simulink model "Simulink_Arduino_PIL_v05"  (R2020a)
settings: Solver=VariableStepAuto  StartTime=0.0  StopTime=Tsim  RelTol=1e-3
values from neighbouring files (symbols this model uses):
  A = [0.637125393971 0.00050275765043 2.56129190029e-05 0.00322036092898 7.22167712685e-07 3.54290406932e-08 0.00050275765043 0.637125393971 -2.56129190029e-05 7.22167712685e-07 0.00322036092898 -3.54290406932e-08 ... (36 elements, 6x6)]    [exitationData.mat]    (also in main_Simulink_Arduino_PIL_v05.m = sys_dt.A; main_Simulink_Arduino_PIL_v05_v2.m = SSDClip.A; result_data.mat = [0.828490331528 0.231089081296 -0.073917292718 -0.1174239001)
  Ac = [-112.5 0 0 1 0 0 0 -112.5 0 0 1 0 ... (36 elements, 6x6)]    [exitationData.mat]    (also in main_Simulink_Arduino_PIL_v05.m = linsys1.A; main_Simulink_Arduino_PIL_v05_v2.m = sys_ct.A; result_data.mat = [-27.8072490393 38.7615323826 -12.4282188209 -19.7589667718 )
  B = [4.02545116123  0.000902709640856; 0.000902709640856  4.02545116123; 4.42863008665e-05  -4.42863008665e-05; 0.00865368892238  9.43336560833e-07; 9.43336560833e-07  0.00865368892238; 4.52711458174e-08  -4.52711458174e-08]    [exitationData.mat]    (also in main_Simulink_Arduino_PIL_v05.m = sys_dt.B; main_Simulink_Arduino_PIL_v05_v2.m = SSDClip.B; result_data.mat = [2.56829781679  3.43071743834; -4.76154072904  -4.0866307491)
  Bc = [1250  0; 0  1250; 0  0; 0  0; 0  0; 0  0]    [exitationData.mat]    (also in main_Simulink_Arduino_PIL_v05.m = linsys1.B; main_Simulink_Arduino_PIL_v05_v2.m = sys_ct.B; result_data.mat = [429.723017402  565.379444728; -795.881801648  -708.39184256)
  C = [0.5  0.5  0  0  0  0; 0  0  0  0  0  -1]    [exitationData.mat]    (also in main_Simulink_Arduino_PIL_v05.m = sys_dt.C; main_Simulink_Arduino_PIL_v05_v2.m = SSDClip.C; result_data.mat = [0.284296065909  -0.589150784937  0.0969360429014  -0.011889)
  Cc = [0.5  0.5  0  0  0  0; 0  0  0  0  0  -1]    [exitationData.mat]    (also in main_Simulink_Arduino_PIL_v05.m = linsys1.C; main_Simulink_Arduino_PIL_v05_v2.m = sys_ct.C; result_data.mat = [0.284296065909  -0.589150784937  0.0969360429014  -0.011889)
  controller = 3    [main_Simulink_Arduino_PIL_v05_v2.m]    (also in result_data.mat)
  Cs = [Cs1 ... (first row only)    [main_Simulink_Arduino_PIL_v05_v2.m]    (also in result_data.mat = [40  0  0  0  0  0; 0  0  0  10  0  0])
  du1 = 0    [exitationData.mat]    (also in main_Simulink_Arduino_PIL_v05.m; main_Simulink_Arduino_PIL_v05_v2.m; result_data.mat)
  du2 = 0    [exitationData.mat]    (also in main_Simulink_Arduino_PIL_v05.m; main_Simulink_Arduino_PIL_v05_v2.m; result_data.mat)
  du_freq1 = 31.4159265359    [exitationData.mat]    (also in main_Simulink_Arduino_PIL_v05.m = 6.28318530718; main_Simulink_Arduino_PIL_v05_v2.m; result_data.mat)
  du_freq2 = 31.4159265359    [exitationData.mat]    (also in main_Simulink_Arduino_PIL_v05.m = 3.14159265359; main_Simulink_Arduino_PIL_v05_v2.m; result_data.mat)
  du_offset1 = 1.57079632679    [exitationData.mat]    (also in main_Simulink_Arduino_PIL_v05.m; main_Simulink_Arduino_PIL_v05_v2.m; result_data.mat)
  du_offset2 = 0    [exitationData.mat]    (also in main_Simulink_Arduino_PIL_v05.m; main_Simulink_Arduino_PIL_v05_v2.m; result_data.mat)
  F = Phi'*QN*Lambda    [MPC_matrices.m]    (also in exitationData.mat = [-0.000573649565694  -0.0645157742088  -9.07938273169  2.078; main_Simulink_Arduino_PIL_v05.m = place(A, B, Pz); main_Simulink_Arduino_PIL_v05_v2.m = dlqr(A,B,Q,R); result_data.mat = [0.00876577681444  -0.0192523630926  0.00317713769136  -0.00)
  G = 300    [Model_2i2o.m]    (also in exitationData.mat; main_Simulink_Arduino_PIL_v05.m; main_Simulink_Arduino_PIL_v05_v2.m = 30; result_data.mat = 30)
  Keq = (Cs*B)^-1 * Cs*A    [main_Simulink_Arduino_PIL_v05_v2.m]    (also in result_data.mat = [0.178878322359  0.0678089646259  -0.00767386477751  -0.0788)
  Ksw = gamma*(Cs*B)^1    [main_Simulink_Arduino_PIL_v05_v2.m]    (also in result_data.mat = [1.02731912671  1.37228697534; -0.365616898703  0.4987768181)
  L = [0  0  0  0  0  0; 0  0  0  0  0  0]    [exitationData.mat]    (also in main_Simulink_Arduino_PIL_v05.m = zeros(2,6); main_Simulink_Arduino_PIL_v05_v2.m = zeros(2,6); result_data.mat = [4.28174074557e-08  8.22289952927e-07; -2.58319761267e-07  3)
  obs = 0    [exitationData.mat]    (also in main_Simulink_Arduino_PIL_v05.m; main_Simulink_Arduino_PIL_v05_v2.m = 2; result_data.mat = 2)
  PIL = 0    [exitationData.mat]    (also in main_Simulink_Arduino_PIL_v05.m; main_Simulink_Arduino_PIL_v05_v2.m = 1; result_data.mat = 1)
  Ts = 1/fs    (= 0.01)    [Model_2i2o.m]    (also in SystemIdentification.m = 0.001; exitationData.mat = 0.001; main_Simulink_Arduino_PIL_v05.m = 0.004; main_Simulink_Arduino_PIL_v05_v2.m)
  uss = Nu*y_star    [main_Simulink_Arduino_PIL_v05_v2.m]    (also in result_data.mat = [8.74234545194 9.2576545493])
  xo_hat = [0 0 0 0 0 0]    [exitationData.mat]    (also in main_Simulink_Arduino_PIL_v05.m = [0 0 0 0 0 0]'; main_Simulink_Arduino_PIL_v05_v2.m = [0 0 0 0 0 0]'; result_data.mat)
  xss = xss    [main_Simulink_Arduino_PIL_v05_v2.m]    (also in result_data.mat = [96.5348220502 72.99080423 1182.48935996 48.3465128204 -17.6)
  z_hat_o = [O1_dot_o, O2_dot_o, x_dot_o]'    [SystemIdentification.m]    (also in exitationData.mat = [100 100 0]; main_Simulink_Arduino_PIL_v05.m; main_Simulink_Arduino_PIL_v05_v2.m; result_data.mat = [0 0 0])
  zo = [O1_o, O2_o, x_o]'    [SystemIdentification.m]    (also in exitationData.mat = [0 0 0.02]; main_Simulink_Arduino_PIL_v05.m; main_Simulink_Arduino_PIL_v05_v2.m = [O1_o, O2_o, -x_o]'; result_data.mat = [0 0 0])
undefined symbols (not defined in the file or in its folder): serial
libraries: instrumentlib x3, simulink x2
settings Model: SimulationMode=accelerator  EnablePacing=on  Creator=ricardo  LastModifiedBy=alastairbate
settings DataIOCC: ReturnWorkspaceOutputs=off
settings DebuggingCC: ArithmeticOperatorsInVariantConditions=warning
settings SFSimCC: CustomCodeUndefinedFunction=UseInterfaceOnly

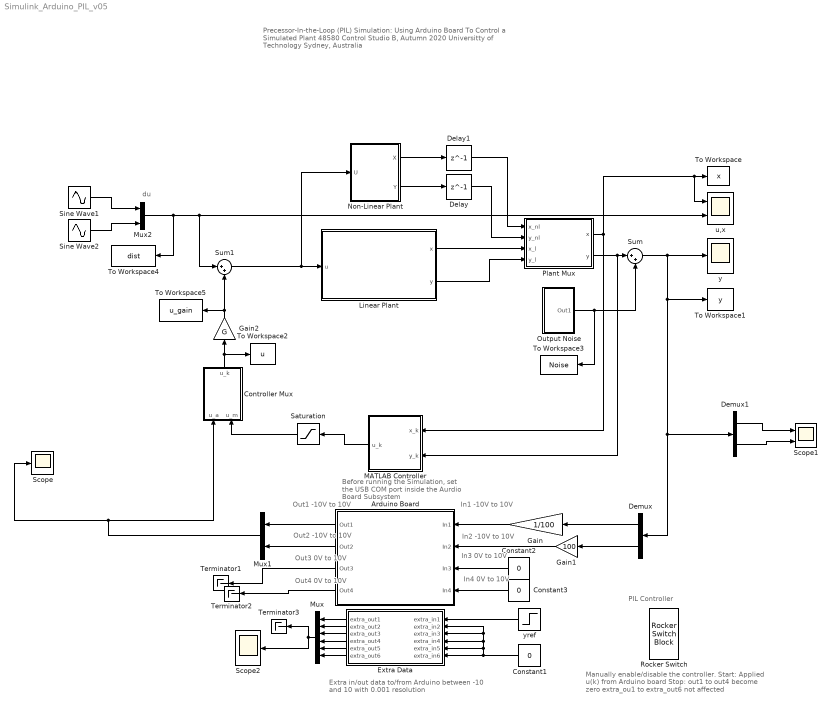
== system Simulink_Arduino_PIL_v05 ==
  note: Out1
      | -10V to 10V
  note: Precessor-In-the-Loop (PIL) Simulation:
      | Using Arduino Board To Control a Simulated Plant
      |
      | 48580 Control Studio B, Autumn 2020
      | Universitty of Technology Sydney, Australia
  note: Out2
      | -10V to 10V
  note: Out3
      | 0V to 10V
  note: Out4
      | 0V to 10V
  note: In1
      | -10V to 10V
  note: In2
      | -10V to 10V
  note: In3
      | 0V to 10V
  note: In4
      | 0V to 10V
  note: Before running the Simulation, set the USB COM port inside the Aurdio Board Subsystem
  note: PIL Controller
  note: Manually enable/disable the controller.
      | Start: Applied u(k) from Arduino board
      | Stop: out1 to out4 become zero
      | extra_ou1 to extra_out6 not affected
  note: Extra in/out data to/from Arduino between -10 and 10 with 0.001 resolution
  note: du
  Arduino Board : Subsystem
      mask Display: image('$imagefile'); % Use "Edit Image" on toolstrip to change.
  Constant1 : Constant  Value=0
  Constant2 : Constant  Value=0
  Constant3 : Constant  Value=0
  Controller Mux : MATLAB Function  TreatAsAtomicUnit=on
  Delay : Delay  DelayLength=1  InitialCondition=0
  Delay1 : Delay  DelayLength=1  InitialCondition=0
  Demux : Demux  Outputs=2
  Demux1 : Demux  Outputs=2
  Extra Data : Subsystem
  Gain : Gain  Gain=1/100
  Gain1 : Gain  Gain=100
  Gain2 : Gain  Gain=G
  Linear Plant : Subsystem
  MATLAB Controller : MATLAB Function  TreatAsAtomicUnit=on  SystemSampleTime=Ts
  Mux : Mux  Inputs=6
  Mux1 : Mux  Inputs=2
  Mux2 : Mux  Inputs=2
  Non-Linear Plant : Subsystem
  Output Noise : Subsystem
  Plant Mux : MATLAB Function  TreatAsAtomicUnit=on
  Rocker Switch : RockerSwitchBlock  LabelPosition=Hide
      settings: Values={{'Stop', 'Start'}, [0 1]}
  Saturation : Saturate  UpperLimit=10  LowerLimit=-10
  Scope : Scope
  Scope1 : Scope  NumInputPorts=2
  Scope2 : Scope
  Sine Wave1 : Sin  Amplitude=du1  Frequency=du_freq1  Phase=du_offset1  SampleTime=0
  Sine Wave2 : Sin  Amplitude=du2  Frequency=du_freq2  Phase=du_offset2  SampleTime=0
  Sum : Sum  Inputs=|++
  Sum1 : Sum  Inputs=|++
  Terminator1 : Terminator
  Terminator2 : Terminator
  Terminator3 : Terminator
  To Workspace : ToWorkspace  VariableName=x  SampleTime=Ts/100
  To Workspace1 : ToWorkspace  VariableName=y  SampleTime=Ts/100
  To Workspace2 : ToWorkspace  VariableName=u  SampleTime=Ts/100
  To Workspace3 : ToWorkspace  VariableName=Noise  SampleTime=Ts/100
  To Workspace4 : ToWorkspace  VariableName=dist  SampleTime=Ts/100
  To Workspace5 : ToWorkspace  VariableName=u_gain  SampleTime=Ts/100
  u,x : Scope  NumInputPorts=2
  y : Scope
  yref : Step  Time=5  Before=4  After=-4  SampleTime=0
  wires:
  Arduino Board/2(Out2) -> Mux1/2
  Constant3/1 -> Arduino Board/4(In4)
  Extra Data/1(extra_out1) -> Mux/1
  Extra Data/2(extra_out2) -> Mux/2
  Extra Data/3(extra_out3) -> Mux/3
  Extra Data/4(extra_out4) -> Mux/4
  Mux/1 -> Scope2/1, Terminator3/1
  yref/1 -> Extra Data/1(extra_in1)
  Extra Data/5(extra_out5) -> Mux/5
  Extra Data/6(extra_out6) -> Mux/6
  Constant1/1 -> Extra Data/5(extra_in5), Extra Data/2(extra_in2), Extra Data/3(extra_in3), Extra Data/4(extra_in4), Extra Data/6(extra_in6)
  Arduino Board/1(Out1) -> Mux1/1
  Mux1/1 -> Scope/1, Controller Mux/1(u_a)
  MATLAB Controller/1(u_k) -> Saturation/1
  Saturation/1 -> Controller Mux/2(u_m)
  Linear Plant/1(x) -> Plant Mux/3(x_l)
  Plant Mux/1(x) -> MATLAB Controller/1(x_k), u,x/1, To Workspace/1
  Linear Plant/2(y) -> Plant Mux/4(y_l)
  Gain2/1 -> Sum1/2, To Workspace5/1
  Non-Linear Plant/2(Y) -> Delay/1
  Delay/1 -> Plant Mux/2(y_nl)
  Non-Linear Plant/1(X) -> Delay1/1
  Delay1/1 -> Plant Mux/1(x_nl)
  Constant2/1 -> Arduino Board/3(In3)
  Sine Wave1/1 -> Mux2/1
  Sine Wave2/1 -> Mux2/2
  Mux2/1 -> To Workspace4/1, Sum1/1, u,x/2
  Plant Mux/2(y) -> MATLAB Controller/2(y_k), Sum/1
  Sum/1 -> To Workspace1/1, Demux1/1, Demux/1, y/1
  Output Noise/1(Out1) -> To Workspace3/1, Sum/2
  Sum1/1 -> Non-Linear Plant/1(U), Linear Plant/1(u)
  Controller Mux/1(u_k) -> To Workspace2/1, Gain2/1
  Arduino Board/3(Out3) -> Terminator1/1
  Arduino Board/4(Out4) -> Terminator2/1
  Demux1/1 -> Scope1/1
  Demux1/2 -> Scope1/2
  Gain/1 -> Arduino Board/1(In1)
  Demux/1 -> Gain/1
  Demux/2 -> Gain1/1
  Gain1/1 -> Arduino Board/2(In2)

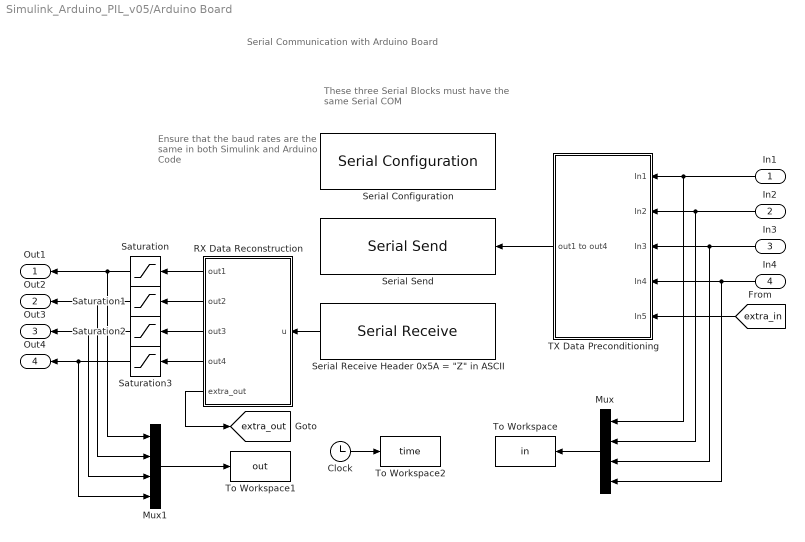
== system Simulink_Arduino_PIL_v05/Arduino Board ==
  note: Ensure that the baud rates are the same in both Simulink and Arduino Code
  note: Serial Communication with Arduino Board
  note: These three Serial Blocks must have the same Serial COM
  In1 : Inport
  In2 : Inport  Port=2
  In3 : Inport  Port=3
  In4 : Inport  Port=4
  Clock : Clock
  Mux : Mux
  Mux1 : Mux
  RX Data Reconstruction : MATLAB Function  TreatAsAtomicUnit=on
  Saturation : Saturate  UpperLimit=10  LowerLimit=-10
  Saturation1 : Saturate  UpperLimit=10  LowerLimit=-10
  Saturation2 : Saturate  UpperLimit=10  LowerLimit=0
  Saturation3 : Saturate  UpperLimit=10  LowerLimit=0
  Serial Configuration : instrumentlib/Serial Configuration  Priority=-200000  ComPortMenu=/dev/cu.usbmodem144301  ComPort=/dev/cu.usbmodem144301  ObjConstructor=serial('/dev/cu.usbmodem144301');  BaudRate=115200  DataBits=8  Parity=none  StopBits=1  FlowControl=none  Timeout=0.0001  ByteOrder=LittleEndian
  "Serial Receive Header 0x5A = \"Z\" in ASCII" : instrumentlib/Serial Receive  ComPortMenu=/dev/cu.usbmodem144301  ComPort=/dev/cu.usbmodem144301  ObjConstructor=serial('/dev/cu.usbmodem144301');  Header=Z  Terminator=<none>  DataSize=21  DataType=uint8  EnableBlockingMode=on  ActionDataUnavailable=Output last received value  CustomValue=0  SampleTime=0.5*Ts
  Serial Send : instrumentlib/Serial Send  ComPortMenu=/dev/cu.usbmodem144301  ComPort=/dev/cu.usbmodem144301  ObjConstructor=serial('/dev/cu.usbmodem144301');  Terminator=<none>  EnableBlockingMode=on
  TX Data Preconditioning : Subsystem
  To Workspace : ToWorkspace  VariableName=in  SampleTime=Ts/20
  To Workspace1 : ToWorkspace  VariableName=out  SampleTime=Ts/20
  To Workspace2 : ToWorkspace  VariableName=time  SampleTime=Ts/100
  Out1 : Outport  VectorParamsAs1DForOutWhenUnconnected=off
  Out2 : Outport  Port=2  VectorParamsAs1DForOutWhenUnconnected=off
  Out3 : Outport  Port=3  VectorParamsAs1DForOutWhenUnconnected=off
  Out4 : Outport  Port=4  VectorParamsAs1DForOutWhenUnconnected=off
  tag scope: extra_out=global
  wires:
  "Serial Receive Header 0x5A = \"Z\" in ASCII"/1 -> RX Data Reconstruction/1(u)
  In1/1 -> TX Data Preconditioning/1(In1), Mux/1
  In2/1 -> TX Data Preconditioning/2(In2), Mux/2
  In3/1 -> TX Data Preconditioning/3(In3), Mux/3
  In4/1 -> TX Data Preconditioning/4(In4), Mux/4
  TX Data Preconditioning/1(out1 to out4) -> Serial Send/1
  RX Data Reconstruction/1(out1) -> Saturation/1
  RX Data Reconstruction/2(out2) -> Saturation1/1
  RX Data Reconstruction/3(out3) -> Saturation2/1
  Mux/1 -> To Workspace/1
  Mux1/1 -> To Workspace1/1
  Clock/1 -> To Workspace2/1
  Saturation/1 -> Out1/1, Mux1/1
  Saturation1/1 -> Out2/1, Mux1/2
  Saturation2/1 -> Out3/1, Mux1/3
  Saturation3/1 -> Out4/1, Mux1/4
  RX Data Reconstruction/4(out4) -> Saturation3/1
  [extra_in] -> TX Data Preconditioning/5(In5)
  RX Data Reconstruction/5(extra_out) -> [extra_out]

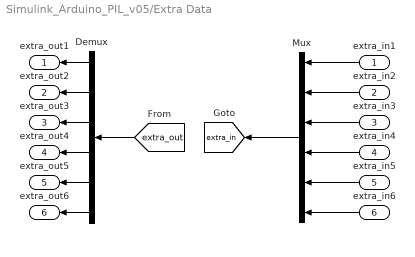
== system Simulink_Arduino_PIL_v05/Extra Data ==
  extra_in1 : Inport
  extra_in2 : Inport  Port=2
  extra_in3 : Inport  Port=3
  extra_in4 : Inport  Port=4
  extra_in5 : Inport  Port=5
  extra_in6 : Inport  Port=6
  Demux : Demux  Outputs=6
  Mux : Mux  Inputs=6
  extra_out1 : Outport
  extra_out2 : Outport  Port=2
  extra_out3 : Outport  Port=3
  extra_out4 : Outport  Port=4
  extra_out5 : Outport  Port=5
  extra_out6 : Outport  Port=6
  tag scope: extra_in=global
  wires:
  extra_in4/1 -> Mux/4
  extra_in3/1 -> Mux/3
  extra_in2/1 -> Mux/2
  extra_in1/1 -> Mux/1
  Mux/1 -> [extra_in]
  [extra_out] -> Demux/1
  Demux/1 -> extra_out1/1
  Demux/2 -> extra_out2/1
  Demux/3 -> extra_out3/1
  Demux/4 -> extra_out4/1
  extra_in5/1 -> Mux/5
  extra_in6/1 -> Mux/6
  Demux/6 -> extra_out6/1
  Demux/5 -> extra_out5/1

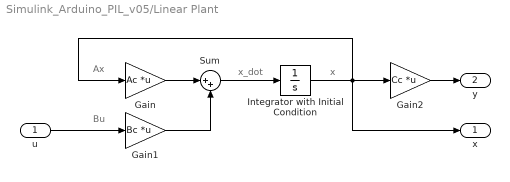
== system Simulink_Arduino_PIL_v05/Linear Plant ==
  note: x
  note: x_dot
  note: Bu
  note: Ax
  u : Inport
  Gain : Gain  Gain=Ac  Multiplication=Matrix(K*u)
  Gain1 : Gain  Gain=Bc  Multiplication=Matrix(K*u)
  Gain2 : Gain  Gain=Cc  Multiplication=Matrix(K*u)
  Integrator with Initial Condition : Integrator
  Sum : Sum  Inputs=|++
  x : Outport  VectorParamsAs1DForOutWhenUnconnected=off
  y : Outport  Port=2  VectorParamsAs1DForOutWhenUnconnected=off
  wires:
  Gain1/1 -> Sum/2
  Sum/1 -> Integrator with Initial Condition/1
  Gain/1 -> Sum/1
  Integrator with Initial Condition/1 -> Gain2/1, x/1, Gain/1
  Gain2/1 -> y/1
  u/1 -> Gain1/1

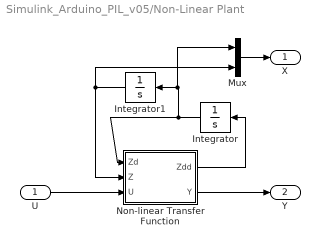
== system Simulink_Arduino_PIL_v05/Non-Linear Plant ==
  U : Inport
  Integrator : Integrator  InitialCondition=z_hat_o
  Integrator1 : Integrator  InitialCondition=zo
  Mux : Mux  Inputs=2
  Non-linear Transfer Function : MATLAB Function  TreatAsAtomicUnit=on
  X : Outport
  Y : Outport  Port=2
  wires:
  Non-linear Transfer Function/2(Y) -> Y/1
  Integrator1/1 -> Mux/2, Non-linear Transfer Function/2(Z)
  Integrator/1 -> Non-linear Transfer Function/1(Zd), Mux/1, Integrator1/1
  Non-linear Transfer Function/1(Zdd) -> Integrator/1
  Mux/1 -> X/1
  U/1 -> Non-linear Transfer Function/3(U)

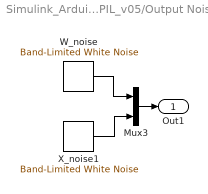
== system Simulink_Arduino_PIL_v05/Output Noise ==
  Mux3 : Mux  Inputs=2
  W_noise : simulink/Sources/Band-Limited White Noise  Cov=w_noise  Ts=0.1  seed=[23341]
  X_noise1 : simulink/Sources/Band-Limited White Noise  Cov=x_noise  Ts=0.1  seed=[23341]
  Out1 : Outport
  wires:
  Mux3/1 -> Out1/1
  X_noise1/1 -> Mux3/2
  W_noise/1 -> Mux3/1

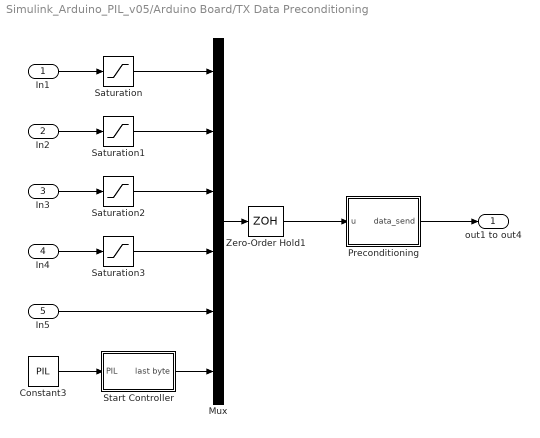
== system Simulink_Arduino_PIL_v05/Arduino Board/TX Data Preconditioning ==
  In1 : Inport
  In2 : Inport  Port=2
  In3 : Inport  Port=3
  In4 : Inport  Port=4
  In5 : Inport  Port=5
  Constant3 : Constant  Value=PIL
  Mux : Mux  Inputs=6
  Preconditioning : MATLAB Function  TreatAsAtomicUnit=on
  Saturation : Saturate  UpperLimit=10  LowerLimit=-10
  Saturation1 : Saturate  UpperLimit=10  LowerLimit=-10
  Saturation2 : Saturate  UpperLimit=10  LowerLimit=0
  Saturation3 : Saturate  UpperLimit=10  LowerLimit=0
  Start Controller : Subsystem
  Zero-Order Hold1 : ZeroOrderHold  SampleTime=Ts
  out1 to out4 : Outport  VectorParamsAs1DForOutWhenUnconnected=off
  wires:
  In1/1 -> Saturation/1
  Preconditioning/1(data_send) -> out1 to out4/1
  Saturation3/1 -> Mux/4
  Saturation2/1 -> Mux/3
  Saturation1/1 -> Mux/2
  In2/1 -> Saturation1/1
  Mux/1 -> Zero-Order Hold1/1
  In4/1 -> Saturation3/1
  In3/1 -> Saturation2/1
  Saturation/1 -> Mux/1
  Zero-Order Hold1/1 -> Preconditioning/1(u)
  In5/1 -> Mux/5
  Constant3/1 -> Start Controller/1(PIL)
  Start Controller/1(last byte) -> Mux/6

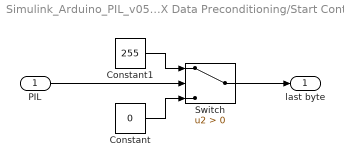
== system Simulink_Arduino_PIL_v05/Arduino Board/TX Data Preconditioning/Start Controller ==
  PIL : Inport
  Constant : Constant  Value=0
  Constant1 : Constant  Value=255
  Switch : Switch  Criteria=u2 > Threshold
  last byte : Outport
  wires:
  Switch/1 -> last byte/1
  PIL/1 -> Switch/2
  Constant1/1 -> Switch/1
  Constant/1 -> Switch/3

== matlab function Simulink_Arduino_PIL_v05/Arduino Board/RX Data Reconstruction ==
  data: u input; out1 output; out2 output; out3 output; out4 output; extra_out output
%% Rx Data from Arduino Board
% 
%
% 48580 Control Studio B,
% The University of Technology Sydney (UTS)
% Sydney, NSW, Australia
%
% Dr Ricardo P. Aguilera
% April 2020
%%%%%%%%%%%%%%%%%%%%%%%%%%%%%%%%%%%%%%%%%%%%%%%%%%%%%%%%%%%%%%%%%%%%%%%%%%%%

function [out1, out2, out3, out4, extra_out] = fcn(u)
N_data=10;


out=zeros(N_data,1);
extra_out=zeros(6,1);

for k=1:N_data
    %% Reconstructing out1
    MSB_uint8 = u(2*k-1); % Least Significant Bits (8 bits)
    LSB_uint8 = u(2*k);  % Most Significant Bits (8 bits)

    % Transforming MSB_uint8 in 16 bits. 
    MSB_uint16 = uint16(MSB_uint8);     %  MSB_unit16 = 00000000 | MSB_uint8 
                                                          % MSB_uint8 is stored as LSB in MSB_uint16                                             
                                                          % Therefore, it has to be shifted in 8 positions

    MSB_uint16 =bitshift(MSB_uint16,8); % MSB_unit16 = MSB_uint8 | 00000000
    out1_uint16 = MSB_uint16+ uint16(LSB_uint8);  % out1_uint16 = MSB_uint8 | LSB_uint8

    %Finally, it is transformed in its original float number
    out(k) = double(out1_uint16)*0.001-10;  
end

%% Clear out data at the beginning and when controller is not active
PIL_start = int8(0);
PIL_start = u(21);
if (PIL_start==0)
    for k=1:4
        out(k)=0;
    end
end

out1 = out(1);
out2 = out(2);
out3 = out(3);
out4 = out(4);

extra_out(1)=out(5);
extra_out(2)=out(6);
extra_out(3)=out(7);
extra_out(4)=out(8);
extra_out(5)=out(9);
extra_out(6)=out(10);

== matlab function Simulink_Arduino_PIL_v05/Arduino Board/TX Data Preconditioning/Preconditioning ==
  data: u input; data_send output
%% Tx Data to Arduino Board
% 
%
% 48580 Control Studio B,
% The University of Technology Sydney (UTS)
% Sydney, NSW, Australia
%
% Dr Ricardo P. Aguilera
% April 2020
%%%%%%%%%%%%%%%%%%%%%%%%%%%%%%%%%%%%%%%%%%%%%%%%%%%%%%%%%%%%%%%%%%%%%%%%%%%%

function data_send = fcn(u)
N_data=10;

data_send=uint8(zeros(2*N_data+2,1));   % array of 2 bytes (2 variables of 8 bits) + Header

%Header
data_send(1)=hex2dec('AA');             %0xAA is for send data in this example

for k=1:N_data
    in = u(k);  %Input singal is between -10 to 10

    %% Data preconditioning to be transmitted as bytes

    in_pos = in+10; % to transform it in an unsigned signal between 0 to 20
    in_uint16= uint16(1000*in_pos); % Transforming it in an unsigned integer of 16 bits

    % Now, the 16 bits variable will be divided in 2 8bits variable.
    % in1_uint16 = MSB_uint8 | LSB_uint8
    % 255(dec) = 00000000|11111111 (16 bits)
    LSB_uint8  = uint8(bitand(in_uint16,255));   %Extraxting Least Significant Bits (8 bits)
    MSB_uint8 = uint8(bitshift(in_uint16,-8));    %Extraxting Most Significant Bits (8 bits)

    % Data is now put in an byte array to be transmitted
    data_send(2*k)=MSB_uint8;
    data_send(2*k+1)=LSB_uint8;
end

data_send(2*(N_data+1))=u(N_data+1);

== matlab function Simulink_Arduino_PIL_v05/MATLAB Controller ==
  data: x_k input; y_k input; F parameter; xo_hat parameter; obs parameter; G parameter; u_k output; xss parameter; controller parameter; uss parameter; A parameter; B parameter; C parameter; L parameter; Keq parameter; Ksw parameter; Cs parameter
function u_k = fcn(x_k, y_k, F, xo_hat, obs, G, xss, controller, uss, A, B, C, L,Keq, Ksw, Cs)

%% Initializing block outputs signals
u_k=zeros(2,1);     %Do not delete
x_hat=zeros(6,1);   %Do not delete

%% Use persistent for variables that requiered to be memorised
persistent x_hat_k
if isempty(x_hat_k)
    x_hat_k = xo_hat;
end
x_hat=x_hat_k;

%% State Feedback Controller (SFC) 
if (obs ~= 0)
  x = x_hat;
else
  x = x_k;
end

if (controller == 1 || controller == 2)
  % Calculate control effort
  r = F*xss + uss
  u_k = -F*x + r;
  
end

if(controller == 3)
    
    u_k = -Keq*(x-xss) -Ksw*tanh(Cs*(x-xss));
    
end  
  
  % Update Observer
  x_hat_k = A*x_hat +B*u_k + L*(y_k - C*x_hat);
  
  % Scale down by motor gain
  u_k = u_k/G;
end

== matlab function Simulink_Arduino_PIL_v05/Controller Mux ==
  data: u_a input; u_k output; u_m input; matlabController parameter
function u_k = fcn(u_a, u_m, matlabController)

%Initialise output
u_k=zeros(2,1);

if matlabController == 1
    u_k = u_m;
else
    u_k = u_a;
end

== matlab function Simulink_Arduino_PIL_v05/Plant Mux ==
  data: x_nl input; y_nl input; x_l input; x output; y_l input; linear parameter; y output
function [x,y] = fcn(x_nl, y_nl, x_l, y_l, linear)

%Initialise output
x = zeros(6,1);
y = zeros(2,1);

if linear == 1
    x = x_l;
    y = y_l;
else
    x = x_nl;
    y = y_nl;
end

== matlab function Simulink_Arduino_PIL_v05/Non-Linear Plant/Non-linear Transfer Function ==
  data: Zd input; Z input; U input; Zdd output; Y output
function [Zdd, Y]  = fcn(Zd, Z, U)
%% House keeping
Zdd=zeros(3,1);
Y = zeros(2,1);

%% System Constants
I = 0.0008;
m = 0.35;
r = 0.03;
k = 50;
ko = 200;
b = 0.09;
bo = 0.5;
h = 0.4; %height

% %% Saturate signals
% if (Z(3,1) > 0.05)
%     Z(3,1) = 0.05;
% end
% if (Z(3,1) < -0.05)
%     Z(3,1) = -0.05;
% end


%% Calculate a new alpha
%x as input
x = Z(3,1);

a = atan((h/(h-x))*(sqrt(3)/3));

%% System Matrices
M = [I 0 0;
     0 I 0;
     0 0 m];
 
B = [b 0 0;
     0 b 0;
     0 0 bo];
 
Knl = [1.5*k*r^2, -1.5*k*r^2, -k*r*cos(a);
       -1.5*k*r^2, 1.5*k*r^2, k*r*cos(a);
       -k*r*cos(a), k*r*cos(a), ko+2*k*cos(a)*cos(a)];
   
% Get the right size input   
Ua = [1 0;
      0 1;
      0 0]*U;

Zdd = (M^-1)*Ua - (M^-1)*B*Zd - (M^-1)*Knl*Z;

% Get the output we want
Y = [(Zd(1,1)+Zd(2,1))/2;   % Average for belt speed
     -Z(3,1)];              % Tension
